simulink model "SingleVehicle_HIL"  (R2016b)
settings: Solver=ode4  StartTime=0.0  StopTime=inf  FixedStep=0.01  RelTol=1e-3  EnableMultiTasking=on
undefined symbols (not defined in the file or in its folder): Angular, dpsi, FromPrescan, IdealSensors, Linear, psi, RHSC, RHSCCmdBus, v, wpFollower, y
undefined symbols (not defined in the file): vd
libraries: robotlib x6, sldrtlib x1
(part 2 of 2)

== matlab function SingleVehicle_HIL/VehicleDynamics/PWAVehicleDynamicsModel ==
  data: delta input; dY output; v input; dv output; psi input; dpsi input; veh_struct parameter; ddpsi output; mode output
function [dY, dv, ddpsi, mode] = fcn(delta, v, psi, dpsi, veh_struct)
% persistent K_f K_r b_f b_r alfa_f alfa_r
lf = veh_struct.lf_pwa;
lr = veh_struct.lr_pwa;
m = veh_struct.mass_pwa;
Iz = veh_struct.Iz_pwa;
C_f1 = veh_struct.Cf1_pwa;
C_r1 = veh_struct.Cr1_pwa;
C_f2 = veh_struct.Cf2_pwa;
C_r2 = veh_struct.Cr2_pwa;
C_f3 = veh_struct.Cf3_pwa;
C_r3 = veh_struct.Cr3_pwa;
bf1 = veh_struct.bf1_pwa;
br1 = veh_struct.br1_pwa;
bf2 = veh_struct.bf2_pwa;
br2 = veh_struct.br2_pwa;
bf3 = veh_struct.bf3_pwa;
br3 = veh_struct.br3_pwa;
f_thre = veh_struct.f_thre_pwa;
r_thre = veh_struct.r_thre_pwa;
vx = veh_struct.vx_pwa;

K_f = 0;
K_r = 0;
b_f = 0;
b_r = 0;
mode = 0;

alfa_f = (v + dpsi*lf)/vx - delta;
alfa_r = (v - dpsi*lr)/vx;


% if ((-f_thre <= alfa_f) && (alfa_f <= f_thre)) && ((-r_thre<= alfa_r) && (alfa_r <=r_thre))
%     K_f = C_f1;
%     K_r = C_r1;
%     b_f = bf1;
%     b_r = br1;
% else if ((-f_thre <= alfa_f) && (alfa_f <= f_thre)) && (alfa_r <= -r_thre)
%         K_f = C_f1;
%         K_r = C_r2;
%         b_f = bf1;
%         b_r = br2;
%         
%     else if ((-f_thre <= alfa_f) && (alfa_f <= f_thre)) && (alfa_r >= r_thre)
%             K_f = C_f1;
%             K_r = C_r3;
%             b_f = bf1;
%             b_r = br3;
%             
%         else if ((alfa_f <= -f_thre) && ((-r_thre<= alfa_r) && (alfa_r <=r_thre)))
%                 K_f = C_f2;
%                 K_r = C_r1;
%                 b_f = bf2;
%                 b_r = br1;
%                 
%             else if (alfa_f <= -f_thre) && (alfa_r <= -r_thre)
%                     K_f = C_f2;
%                     K_r = C_r2;
%                     b_f = bf2;
%                     b_r = br2;
%                     
%                 else if (alfa_f <= -f_thre) && (alfa_r >= r_thre)
%                         K_f = C_f2;
%                         K_r = C_r3;
%                         b_f = bf2;
%                         b_r = br3;
%                         
%                     else if (alfa_f >= f_thre) && ((-r_thre<= alfa_r) && (alfa_r <=r_thre))
%                             K_f = C_f3;
%                             K_r = C_r1;
%                             b_f = bf3;
%                             b_r = br1;
%                             
%                         else if (alfa_f >= f_thre) && (alfa_r <= -r_thre)
%                                 K_f = C_f3;
%                                 K_r = C_r2;
%                                 b_f = bf3;
%                                 b_r = br2;
%                                 
%                             else if (alfa_f >= f_thre) && (alfa_r >= r_thre)
%                                     K_f = C_f3;
%                                     K_r = C_r3;
%                                     b_f = bf3;
%                                     b_r = br3;
%                                     
%                                 end
%                             end
%                         end
%                     end
%                 end
%             end
%         end
%     end
% end

if ((-r_thre<= alfa_r) && (alfa_r <=r_thre))
    K_f = C_f1;
    K_r = C_r1;
    b_f = bf1;
    b_r = br1;
    mode = 1;
else if  (alfa_r <= -r_thre)
        K_f = C_f1;
        K_r = C_r2;
        b_f = bf1;
        b_r = br2;
        mode = 2;
    else if  (alfa_r >= r_thre)
            K_f = C_f1;
            K_r = C_r3;
            b_f = bf1;
            b_r = br3;
            mode = 3;
        end
    end
end

dY = vx*psi + v;
dv = (K_f + K_r)/m/vx*v + ((K_f*lf - K_r*lr)/m/vx - vx)*dpsi - K_f/m*delta + (b_f + b_r)/m;
ddpsi = (K_f*lf - K_r*lr)/Iz/vx*v + (K_f*lf^2 + K_r*lr^2)/Iz/vx*dpsi - K_f*lf/Iz*delta + (b_f*lf - b_r*lr)/Iz;

== matlab function SingleVehicle_HIL/Subsystem/Actuation/DynamicControls ==
  data: ActReq input Bus: ArbitratedActuationReq; Ctl input Bus: ControllerMainBus; ActCmds output Bus: ActuationCmdBus; ActCmdsPrev input Bus: ActuationCmdBus
function ActCmds  = fcn(ActReq, Ctl, ActCmdsPrev)

v_des = ActReq.v_des;
a_des = ActReq.a_des;
psi_des = ActReq.psi_des;
dpsi_des = ActReq.dpsi_des;

% ActCmds = ActCmdsPrev;
% ActCmds.accel_cmd = 0;
% ActCmds.decel_cmd = 0;
% ActCmds.steering_cmd = 0.1;

ActCmds = ActCmdsPrev;

if a_des >= 0
    ActCmds.accel_cmd = ActReq.a_des;
    ActCmds.decel_cmd = 0;
else
    ActCmds.accel_cmd = 0;
    ActCmds.decel_cmd = ActReq.a_des;
end

psi_des = unwrap(psi_des);
Ctl.IdealSensors.psi = unwrap(Ctl.IdealSensors.psi);

% ActCmds.steering_cmd = 3.5*(psi_des - Ctl.IdealSensors.psi);
ActCmds.steering_cmd = Ctl.FunctionFeatures.RHSCCmdBus.RHSC_steering_cmd;

== matlab function SingleVehicle_HIL/Subsystem/CtlMainBusUnitDelayAndInit/MATLAB Function ==
  data: u input; y output Bus: ControllerMainBus; veh_struct parameter
function y = DelayAndInitCtlBus(u, veh_struct)
coder.extrinsic('exist')
persistent a

y0 = struct;

y0.ActuationCmdBus = struct;
y0.ActuationCmdBus.steering_cmd = 0;
y0.ActuationCmdBus.decel_cmd = 0;
y0.ActuationCmdBus.accel_cmd = 0;



y0.ArbitratedActuationReq = struct;
y0.ArbitratedActuationReq.RHSCCmdBus = struct;
y0.ArbitratedActuationReq.RHSCCmdBus.RHSC_steering_cmd = 0;
y0.ArbitratedActuationReq.v_des = 0;
y0.ArbitratedActuationReq.a_des = 0;
y0.ArbitratedActuationReq.psi_des = 0;
y0.ArbitratedActuationReq.dpsi_des = 0;



y0.FunctionFeatures = struct;
y0.FunctionFeatures.RHSCCmdBus = struct;
y0.FunctionFeatures.RHSCCmdBus.RHSC_steering_cmd = 0;
y0.FunctionFeatures.wpFollower = struct;
y0.FunctionFeatures.wpFollower.v_des = 0;
y0.FunctionFeatures.wpFollower.a_des = 0;
y0.FunctionFeatures.wpFollower.psi_des = 0;
y0.FunctionFeatures.wpFollower.dpsi_des = 0;



y0.situationBus = struct;
y0.situationBus.wP = struct;

y0.situationBus.wP.finalWayPoint = struct;
y0.situationBus.wP.finalWayPoint.x = 0;
y0.situationBus.wP.finalWayPoint.y = 0;
y0.situationBus.wP.finalWayPoint.z = 0;
y0.situationBus.wP.finalWayPoint.treach = 0;

y0.situationBus.wP.currentWayPoint = struct;
y0.situationBus.wP.currentWayPoint.x = 0;
y0.situationBus.wP.currentWayPoint.y = 0;
y0.situationBus.wP.currentWayPoint.z = 0;
y0.situationBus.wP.currentWayPoint.treach = 0;

y0.situationBus.wP.finalWayPointIndex = uint16(1);
y0.situationBus.wP.currentWayPointIndex = uint16(10);

%y0.situationBus.wP.wayPointArray = struct;
wPArray = struct;
wPArray.x = 0;
wPArray.y = 0;
wPArray.z = 0;
wPArray.treach = 0;
y0.situationBus.wP.wayPointArray = repmat(wPArray,100,1);


y0.situationBus.selfAwarenessBus = struct;
y0.situationBus.selfAwarenessBus.x = 0;
y0.situationBus.selfAwarenessBus.y = 0;
y0.situationBus.selfAwarenessBus.z = 0;
y0.situationBus.selfAwarenessBus.theta = 0;
y0.situationBus.selfAwarenessBus.phi = 0;
y0.situationBus.selfAwarenessBus.psi = 0;
y0.situationBus.selfAwarenessBus.u = 0;
y0.situationBus.selfAwarenessBus.v = 0;
y0.situationBus.selfAwarenessBus.w = 0;
y0.situationBus.selfAwarenessBus.dtheta = 0;
y0.situationBus.selfAwarenessBus.dphi = 0;
y0.situationBus.selfAwarenessBus.dpsi = 0;
y0.IdealSensors = struct;
y0.IdealSensors.x = 0;
y0.IdealSensors.y = 0;
y0.IdealSensors.z = 0;
y0.IdealSensors.theta = 0;
y0.IdealSensors.phi = 0;
y0.IdealSensors.psi = 0;
y0.IdealSensors.u = 0;
y0.IdealSensors.v = 0;
y0.IdealSensors.w = 0;
y0.IdealSensors.dtheta = 0;
y0.IdealSensors.dphi = 0;
y0.IdealSensors.dpsi = 0;
y0.FromPrescan = struct;
y0.FromPrescan.x = 0;
y0.FromPrescan.y = 0;
y0.FromPrescan.z = 0;
y0.FromPrescan.Rotx = 0;
y0.FromPrescan.Roty = 0;
y0.FromPrescan.Rotz = 0;
y0.FromPrescan.GPS_lat = 0;
y0.FromPrescan.GPS_long = 0;
y0.FromPrescan.u = 0;
y0.FromPrescan.GPS_alt = 0;
y0.FromPrescan.heading = 0;
y0.FromPrescan.Yaw_rate = 0;



if isempty(a)
    a = 1;
    y = y0;
    y.situationBus.wP.wayPointArray = veh_struct.initialWayPointsArray;
    y.situationBus.wP.currentWayPointIndex = veh_struct.initialCurrentWayPointIndex;
    y.situationBus.wP.finalWayPointIndex = veh_struct.initialFinalWayPointIndex;

else
    y = u;
end

== matlab function SingleVehicle_HIL/Subsystem/FeaturedFunctions/wpFollower ==
  data: prevWpAction input Bus: wpFollower; prevSituation input Bus: situationBus; wpAction output Bus: wpFollower; veh_struct parameter; newSituation output Bus: situationBus
function [wpAction, newSituation] = wpFollower(prevWpAction, prevSituation, veh_struct)

currentIndex = prevSituation.wP.currentWayPointIndex;
if currentIndex < 1
    currentIndex = uint16(1);
end
finalIndex = prevSituation.wP.finalWayPointIndex;

xd = prevSituation.wP.wayPointArray(currentIndex).x;
yd = prevSituation.wP.wayPointArray(currentIndex).y;
xa = prevSituation.selfAwarenessBus.x;
ya = prevSituation.selfAwarenessBus.y;
howClose = norm([xd-xa, yd-ya]);

if howClose < veh_struct.wpControl.wayPointThreshold
    if (currentIndex == finalIndex)
        currentIndex = uint16(1);
    else
        currentIndex = uint16(currentIndex + 1);
    end
end

newSituation = prevSituation;
newSituation.wP.currentWayPointIndex = uint16(currentIndex);
newSituation.wP.currentWayPoint.x = newSituation.wP.wayPointArray(currentIndex).x;
newSituation.wP.currentWayPoint.y = newSituation.wP.wayPointArray(currentIndex).y;
newSituation.wP.currentWayPoint.z = newSituation.wP.wayPointArray(currentIndex).z;
newSituation.wP.currentWayPoint.treach = newSituation.wP.wayPointArray(currentIndex).treach;

v_des_raw = min(veh_struct.wpControl.v_des_max, howClose / veh_struct.wpControl.howClose_saturate * veh_struct.wpControl.v_des_max);
psi_des_raw = atan2((yd-ya),(xd-xa));

% if psi_des_raw < 0
%     
%     dbg = 1;
%     
% end
    

v_des_old = prevWpAction.v_des;
psi_des_old = prevWpAction.psi_des;

a_des = veh_struct.wpControl.v_des_filter.lambda * (v_des_raw - v_des_old);
v_des = v_des_old + veh_struct.CONTROL_OS_SAMPLETIME * a_des;

dpsi_des = veh_struct.wpControl.psi_des_filter.lambda * (psi_des_raw - psi_des_old);
psi_des = psi_des_old + veh_struct.CONTROL_OS_SAMPLETIME * dpsi_des;
% psi_des = mod(psi_des, 2 * pi);


wpAction.v_des = v_des;
wpAction.a_des = a_des;
wpAction.psi_des = psi_des;
wpAction.dpsi_des = dpsi_des;

end

== matlab function SingleVehicle_HIL/Subsystem/SituationalAwareness/situationAwareness ==
  data: prevSituation input Bus: situationBus; newSituation output Bus: situationBus; prescanSimData input Bus: PrescanSimData; idealSensors input Bus: VehState; veh_struct parameter
function newSituation = calcSituationAwareness(prevSituation,prescanSimData,idealSensors, veh_struct)

newSituation = prevSituation;


newSituation.selfAwarenessBus.x = idealSensors.x;
newSituation.selfAwarenessBus.y = idealSensors.y;
newSituation.selfAwarenessBus.z = idealSensors.z;
newSituation.selfAwarenessBus.theta = idealSensors.theta;
newSituation.selfAwarenessBus.phi = idealSensors.phi;
newSituation.selfAwarenessBus.psi = idealSensors.psi;
newSituation.selfAwarenessBus.u = idealSensors.u;
newSituation.selfAwarenessBus.v = idealSensors.v;
newSituation.selfAwarenessBus.w = idealSensors.w;
newSituation.selfAwarenessBus.dtheta = idealSensors.dtheta;
newSituation.selfAwarenessBus.dphi = idealSensors.dphi;
newSituation.selfAwarenessBus.dpsi = idealSensors.dpsi;

end

== matlab function SingleVehicle_HIL/Subsystem/StrategicArbitration/Arbitration ==
  data: FunctionFeatures input Bus: FunctionFeatures; ArbitratedReq output Bus: ArbitratedActuationReq
function ArbitratedReq = Arbitrate(FunctionFeatures)

ArbitratedReq.RHSCCmdBus.RHSC_steering_cmd = FunctionFeatures.RHSCCmdBus.RHSC_steering_cmd;
ArbitratedReq.v_des = FunctionFeatures.wpFollower.v_des;
ArbitratedReq.a_des = FunctionFeatures.wpFollower.a_des;
ArbitratedReq.psi_des = FunctionFeatures.wpFollower.psi_des;
ArbitratedReq.dpsi_des = FunctionFeatures.wpFollower.dpsi_des;



end
